simulink model "OFDM_Rx_HW"  (R2020a)
settings: Solver=FixedStepDiscrete  StartTime=0.0  StopTime=inf  RelTol=1e-3
PostLoadFcn:
  | run ./scripts/filter_setup;
InitFcn:
  | % Set parameters
  | fs = 1e6;
  | 
  | % Load all required variables
  | load('variables/read_addr_data');
  | load('variables/read_addr_cp');
  | load('variables/read_addr_pream');
  | load('variables/read_addr_rx');
  | load('variables/pilot');
  | load('variables/sc_index');
  | load('variables/LTSfreq');
  | load('variables/STSfreq');
  | load('variables/LTSread');
  | load('variables/STSread');
undefined symbols (not defined in the file): CIC_fine_Tx
libraries: hdlsllib x11, dspmlti4 x4, xbsIndex_r4 x1, lib_decimaterx x1, lib_ofdmrx x1, lib_ofdmtx x1
settings Model: SimulationMode=accelerator  Creator=njb13206  LastModifiedBy=LDM
settings OptimizationCC: BlockReduction=off  ConditionallyExecuteInputs=off  DefaultParameterBehavior=Inlined
settings DebuggingCC: AlgebraicLoopMsg=error  IntegerOverflowMsg=none  ParameterPrecisionLossMsg=none  IntegerSaturationMsg=none
settings HardwareCC: ProdBitPerPointer=32  ProdBitPerSizeT=32  ProdBitPerPtrDiffT=32  ProdLargestAtomicFloat=None  ProdIntDivRoundTo=Undefined  ProdEndianess=Unspecified  ProdWordSize=32  ProdHWDeviceType=ASIC/FPGA->ASIC/FPGA  TargetBitPerPointer=64  TargetBitPerSizeT=64  TargetBitPerPtrDiffT=64  TargetLongLongMode=on  TargetIntDivRoundTo=Zero  TargetEndianess=LittleEndian  TargetWordSize=64  TargetHWDeviceType=Custom Processor->MATLAB Host Computer  ProdEqTarget=off

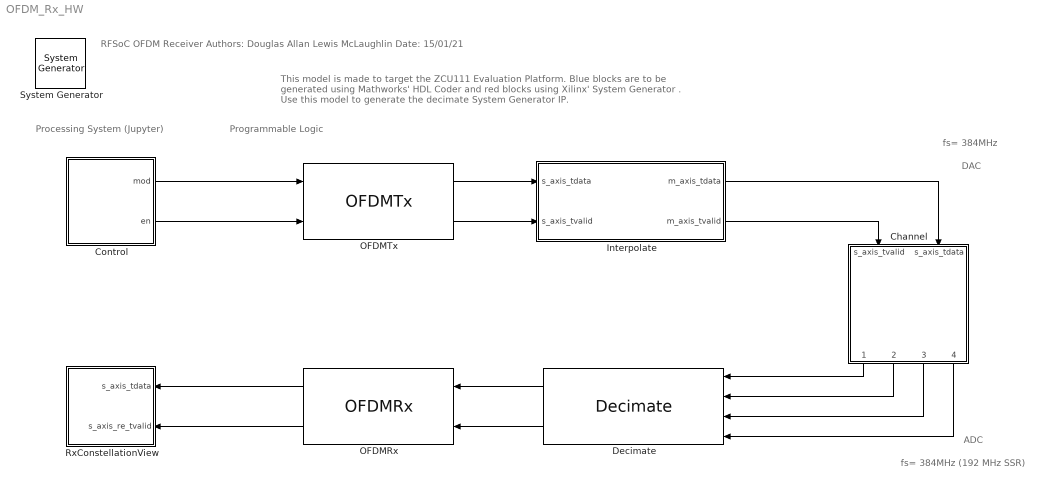
== system OFDM_Rx_HW ==
  note: This model is made to target the ZCU111 Evaluation Platform. Blue blocks are to be generated using Mathworks' HDL Coder and red blocks using Xilinx' System Generator .
      |
      | Use this model to generate the decimate System Generator IP.
  note: Programmable Logic
  note: Processing System (Jupyter)
  note: DAC
  note: fs= 384MHz
  note: ADC
  note: fs= 384MHz (192 MHz SSR)
  note: RFSoC OFDM Receiver
      | Authors: Douglas Allan
      | Lewis McLaughlin
      | Date: 15/01/21
  " System Generator" : xbsIndex_r4/ System Generator  Tag=genX  xilinxfamily=zynquplusRFSOC  part=xczu28dr  speed=-2-e  package=ffvg1517  synthesis_tool=Vivado  clock_wrapper=Clock Enables  directory=C:/Git/rfsoc_ofdm_workspace/models/sys_prj/rx  proj_type=Vivado  Synth_file=Vivado Synthesis Defaults  Impl_file=Vivado Implementation Defaults  testbench=off  simulink_period=1/192e6  sysclk_period=1000/192  dcm_input_clock_period=10  incr_netlist=off  trim_vbits=Everywhere in SubSystem  dbl_ovrd=According to Block Masks  core_generation=According to Block Masks  run_coregen=off  deprecated_control=off  eval_field=0  block_type=sysgen
  Channel : Subsystem
  Control : Subsystem  mask{mod_mask=32QAM, en=on}
      mask prompts: mod_mask "Modulation"; en "Enable"
      mask init:
      | % RF Signal Generator
      | if strcmpi(get_param(gcb, 'mod_mask'), 'BPSK')
      |     mod = 0;
      | elseif strcmpi(get_param(gcb, 'mod_mask'), 'QPSK')
      |     mod = 1;
      | elseif strcmpi(get_param(gcb, 'mod_mask'), '8PSK')
      |     mod = 2;
      | elseif strcmpi(get_param(gcb, 'mod_mask'), '16QAM')
      |     mod = 3;
      | elseif strcmpi(get_param(gcb, 'mod_mask'), '32QAM')
      |     mod = 4;
      | elseif strcmpi(get_param(gcb, 'mod_mask'), '64QAM')
      |     mod = 5;
      | elseif strcmpi(get_param(gcb, 'mod_mask'), '128QAM')
      |     mod = 6;
      | elseif strcmpi(get_param(gcb, 'mod_mask'), '256QAM')
      |     mod = 7;
      | elseif strcmpi(get_param(gcb, 'mod_mask'), '512QAM')
      |     mod = 8;
      | elseif strcmpi(get_param(gcb, 'mod_mask'), '1024QAM')
      |     mod = 9;
      | end
      mask TypeOptions mod_mask: BPSK | QPSK | 8PSK | 16QAM | 32QAM | 64QAM | 128QAM | 256QAM | 512QAM | 1024QAM
      mask DialogControl DescGroupVar Prompt: RF Signal Generator
      mask DialogControl DescTextVar Prompt: Exposes parameters the user can control from Jupyter when running on the target.
      mask DialogControl Container3 Prompt: Control
  Decimate : lib_decimaterx/Decimate  SystemSampleTime=-1  Latency=0  AutoFrameSizeCalculation=off
      link override Up Sample2: sample_ratio=12  copy_samples=off  en=off  latency=1  dbl_ovrd=off
      link override Up Sample2: infoedit="Up samples input data.  Inserted values  can be zeros or copies of the most recent input sample.<br><br>Hardware notes: No hardware is needed if inserted values are copies of the input sample; otherwise, a mux and single bit flip-flop are used."
  Interpolate : Subsystem
  OFDMRx : lib_ofdmrx/OFDMRx  SystemSampleTime=-1  Latency=0  AutoFrameSizeCalculation=off
  OFDMTx : lib_ofdmtx/OFDMTx  SystemSampleTime=-1  Latency=0  AutoFrameSizeCalculation=off
  RxConstellationView : Subsystem
  wires:
  OFDMTx/1 -> Interpolate/1(s_axis_tdata)
  OFDMTx/2 -> Interpolate/2(s_axis_tvalid)
  Channel/1(m00_axis_re_tdata) -> Decimate/1
  Channel/3(m01_axis_im_tdata) -> Decimate/3
  Channel/4(m_axis_im_tvalid) -> Decimate/4
  Channel/2(m_axis_re_tvalid) -> Decimate/2
  Interpolate/1(m_axis_tdata) -> Channel/2(s_axis_tdata)
  Interpolate/2(m_axis_tvalid) -> Channel/1(s_axis_tvalid)
  OFDMRx/2 -> RxConstellationView/2(s_axis_re_tvalid)
  Decimate/1 -> OFDMRx/1
  Decimate/2 -> OFDMRx/2
  OFDMRx/1 -> RxConstellationView/1(s_axis_tdata)
  Control/1(mod) -> OFDMTx/1
  Control/2(en) -> OFDMTx/2

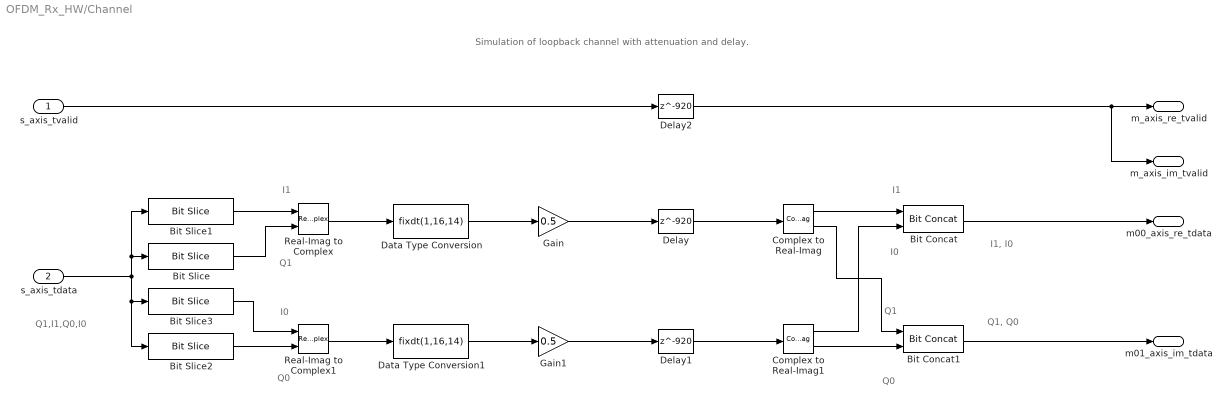
== system OFDM_Rx_HW/Channel ==
  note: Q1, Q0
  note: I1, I0
  note: Q0
  note: I0
  note: Q1
  note: I1
  note: Q1,I1,Q0,I0
  note: Simulation of loopback channel with attenuation and delay.
  note: I1
  note: I0
  note: Q1
  note: Q0
  s_axis_tvalid : Inport
  s_axis_tdata : Inport  Port=2
  Bit Concat : hdlsllib/Logic and Bit Operations/Bit Concat  numInputs=2
  Bit Concat1 : hdlsllib/Logic and Bit Operations/Bit Concat  numInputs=2
  Bit Slice : hdlsllib/Logic and Bit Operations/Bit Slice  lidx=63  ridx=48
      settings: SourceProductBaseCode=SL
  Bit Slice1 : hdlsllib/Logic and Bit Operations/Bit Slice  lidx=47  ridx=32
      settings: SourceProductBaseCode=SL
  Bit Slice2 : hdlsllib/Logic and Bit Operations/Bit Slice  lidx=31  ridx=16
      settings: SourceProductBaseCode=SL
  Bit Slice3 : hdlsllib/Logic and Bit Operations/Bit Slice  lidx=15  ridx=0
      settings: SourceProductBaseCode=SL
  Complex to Real-Imag : ComplexToRealImag
  Complex to Real-Imag1 : ComplexToRealImag
  Data Type Conversion : DataTypeConversion  OutDataTypeStr=fixdt(1,16,14)  ConvertRealWorld=Stored Integer (SI)
  Data Type Conversion1 : DataTypeConversion  OutDataTypeStr=fixdt(1,16,14)  ConvertRealWorld=Stored Integer (SI)
  Delay : Delay  DelayLength=920
  Delay1 : Delay  DelayLength=920
  Delay2 : Delay  DelayLength=920
  Gain : Gain  Gain=0.5  ParamDataTypeStr=double  OutDataTypeStr=fixdt(1,16,14)
  Gain1 : Gain  Gain=0.5  ParamDataTypeStr=double  OutDataTypeStr=fixdt(1,16,14)
  Real-Imag to Complex : RealImagToComplex
  Real-Imag to Complex1 : RealImagToComplex
  m00_axis_re_tdata : Outport  VectorParamsAs1DForOutWhenUnconnected=off
  m_axis_re_tvalid : Outport  Port=2  VectorParamsAs1DForOutWhenUnconnected=off
  m01_axis_im_tdata : Outport  Port=3  VectorParamsAs1DForOutWhenUnconnected=off
  m_axis_im_tvalid : Outport  Port=4  VectorParamsAs1DForOutWhenUnconnected=off
  wires:
  Gain/1 -> Delay/1
  s_axis_tvalid/1 -> Delay2/1
  Delay/1 -> Complex to Real-Imag/1
  Delay2/1 -> m_axis_im_tvalid/1, m_axis_re_tvalid/1
  s_axis_tdata/1 -> Bit Slice1/1, Bit Slice/1, Bit Slice2/1, Bit Slice3/1
  Delay1/1 -> Complex to Real-Imag1/1
  Gain1/1 -> Delay1/1
  Bit Slice/1 -> Real-Imag to Complex/2
  Bit Slice1/1 -> Real-Imag to Complex/1
  Bit Slice2/1 -> Real-Imag to Complex1/2
  Bit Slice3/1 -> Real-Imag to Complex1/1
  Real-Imag to Complex/1 -> Data Type Conversion/1
  Real-Imag to Complex1/1 -> Data Type Conversion1/1
  Complex to Real-Imag1/1 -> Bit Concat/2
  Complex to Real-Imag/1 -> Bit Concat/1
  Complex to Real-Imag1/2 -> Bit Concat1/2
  Complex to Real-Imag/2 -> Bit Concat1/1
  Data Type Conversion/1 -> Gain/1
  Data Type Conversion1/1 -> Gain1/1
  Bit Concat1/1 -> m01_axis_im_tdata/1
  Bit Concat/1 -> m00_axis_re_tdata/1

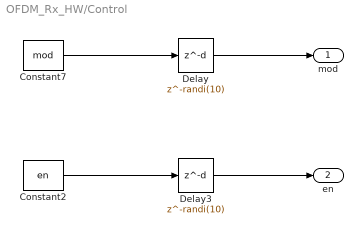
== system OFDM_Rx_HW/Control ==
  Constant2 : Constant  Value=en  OutDataTypeStr=boolean  SampleTime=1/(fs*12)
  Constant7 : Constant  Value=mod  VectorParams1D=off  OutDataTypeStr=uint32  SampleTime=1/(fs*12)
  Delay : Delay  DelayLength=randi(10)
  Delay3 : Delay  DelayLength=randi(10)
  mod : Outport  VectorParamsAs1DForOutWhenUnconnected=off
  en : Outport  Port=2  VectorParamsAs1DForOutWhenUnconnected=off
  wires:
  Delay3/1 -> en/1
  Delay/1 -> mod/1
  Constant7/1 -> Delay/1
  Constant2/1 -> Delay3/1

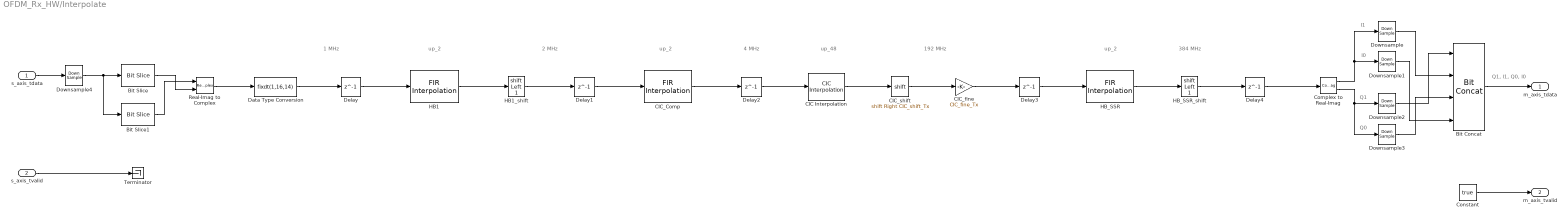
== system OFDM_Rx_HW/Interpolate ==
  note: I0
  note: I1
  note: Q0
  note: Q1
  note: up_2
  note: 4 MHz
  note: 2 MHz
  note: 1 MHz
  note: 384 MHz
  note: 192 MHz
  note: up_2
  note: up_48
  note: up_2
  note: Q1, I1, Q0, I0
  s_axis_tdata : Inport
  s_axis_tvalid : Inport  Port=2
  Bit Concat : hdlsllib/Logic and Bit Operations/Bit Concat  numInputs=4
  Bit Slice : hdlsllib/Logic and Bit Operations/Bit Slice  lidx=15  ridx=0
      settings: SourceProductBaseCode=SL
  Bit Slice1 : hdlsllib/Logic and Bit Operations/Bit Slice  lidx=31  ridx=16
      settings: SourceProductBaseCode=SL
  CIC Interpolation : dspmlti4/CIC Interpolation  filtFrom=Filter object  filtobj=CIC  ftype=Interpolator  R=240  M=1  N=5  filterInternals=Full precision  BPS=[16 16 16 16]  FLPS=0  outputWordLength=32  outputFracLength=0  launchFVT=off  framing=Allow multirate processing  OutputFrames=off
      settings: SourceProductBaseCode=DS
  CIC_Comp : dspmlti4/FIR Interpolation  FilterSource=Dialog parameters  PrivateCoeffs=0  h=WComp.Numerator  L=2  FilterObject=FINTERP  framing=Allow multirate processing  outputBufInitCond=0  roundingMode=Floor  overflowMode=off  firstCoeffMode=Binary point scaling  firstCoeffWordLength=16  firstCoeffFracLength=15  firstCoeffDataTypeStr=fixdt(1,16,15)  firstCoeffMin=[]  firstCoeffMax=[]  firstCoeffLastDataTypeStr=fixdt(1,16,15)  outputMode=Binary point scaling  outputWordLength=16  outputFracLength=14  outputDataTypeStr=fixdt(1,16,14)  outputMin=[]  outputMax=[]  outputLastDataTypeStr=fixdt(1,16,14)
  CIC_fine : Gain  Gain=CIC_fine_Tx  OutDataTypeStr=fixdt(1,16,14)
  CIC_shift : ArithShift  BitShiftNumber=CIC_shift_Tx  BitShiftDirection=Right
  Complex to Real-Imag : ComplexToRealImag
  Constant : Constant  Value=true  SampleTime=2/384e6
  Data Type Conversion : DataTypeConversion  OutDataTypeStr=fixdt(1,16,14)  ConvertRealWorld=Stored Integer (SI)
  Delay{,1..4} (5 alike) : Delay  DelayLength=1
  Downsample : DownSample  phase=1  RateOptions=Allow multirate processing
  Downsample1 : DownSample  RateOptions=Allow multirate processing
  Downsample2 : DownSample  phase=1  RateOptions=Allow multirate processing
  Downsample3 : DownSample  RateOptions=Allow multirate processing
  Downsample4 : DownSample  N=12  phase=5  RateOptions=Allow multirate processing
  HB1 : dspmlti4/FIR Interpolation  FilterSource=Dialog parameters  PrivateCoeffs=0  h=W_HB.Numerator  L=2  FilterObject=FINTERP  framing=Allow multirate processing  outputBufInitCond=0  roundingMode=Floor  overflowMode=off  firstCoeffMode=Binary point scaling  firstCoeffWordLength=16  firstCoeffFracLength=15  firstCoeffDataTypeStr=fixdt(1,16,15)  firstCoeffMin=[]  firstCoeffMax=[]  firstCoeffLastDataTypeStr=fixdt(1,16,15)  outputMode=Binary point scaling  outputWordLength=16  outputFracLength=14  outputDataTypeStr=fixdt(1,16,14)  outputMin=[]  outputMax=[]  outputLastDataTypeStr=fixdt(1,16,14)
  HB1_shift : ArithShift  BitShiftNumber=1  BitShiftDirection=Left
  HB_SSR : dspmlti4/FIR Interpolation  FilterSource=Dialog parameters  PrivateCoeffs=0  h=W_HB_ssr.Numerator  L=2  FilterObject=FINTERP  framing=Allow multirate processing  outputBufInitCond=0  roundingMode=Floor  overflowMode=off  firstCoeffMode=Binary point scaling  firstCoeffWordLength=16  firstCoeffFracLength=15  firstCoeffDataTypeStr=fixdt(1,16,15)  firstCoeffMin=[]  firstCoeffMax=[]  firstCoeffLastDataTypeStr=fixdt(1,16,15)  outputMode=Binary point scaling  outputWordLength=16  outputFracLength=14  outputDataTypeStr=fixdt(1,16,14)  outputMin=[]  outputMax=[]  outputLastDataTypeStr=fixdt(1,16,14)
  HB_SSR_shift : ArithShift  BitShiftNumber=1  BitShiftDirection=Left
  Real-Imag to Complex : RealImagToComplex
  Terminator : Terminator
  m_axis_tdata : Outport
  m_axis_tvalid : Outport  Port=2
  wires:
  CIC_fine/1 -> Delay3/1
  CIC_shift/1 -> CIC_fine/1
  HB_SSR_shift/1 -> Delay4/1
  HB_SSR/1 -> HB_SSR_shift/1
  CIC Interpolation/1 -> CIC_shift/1
  HB1_shift/1 -> Delay1/1
  CIC_Comp/1 -> Delay2/1
  HB1/1 -> HB1_shift/1
  Real-Imag to Complex/1 -> Data Type Conversion/1
  Delay/1 -> HB1/1
  Delay1/1 -> CIC_Comp/1
  Delay2/1 -> CIC Interpolation/1
  Delay3/1 -> HB_SSR/1
  Delay4/1 -> Complex to Real-Imag/1
  Constant/1 -> m_axis_tvalid/1
  Complex to Real-Imag/1 -> Downsample/1, Downsample1/1
  Complex to Real-Imag/2 -> Downsample3/1, Downsample2/1
  Downsample/1 -> Bit Concat/2
  Downsample2/1 -> Bit Concat/1
  Downsample3/1 -> Bit Concat/3
  Downsample1/1 -> Bit Concat/4
  Bit Concat/1 -> m_axis_tdata/1
  s_axis_tvalid/1 -> Terminator/1
  s_axis_tdata/1 -> Downsample4/1
  Downsample4/1 -> Bit Slice1/1, Bit Slice/1
  Bit Slice/1 -> Real-Imag to Complex/2
  Bit Slice1/1 -> Real-Imag to Complex/1
  Data Type Conversion/1 -> Delay/1

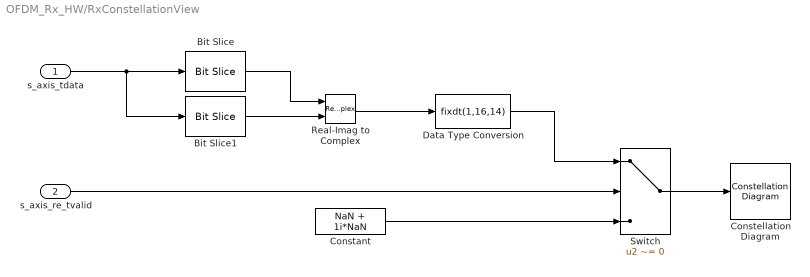
== system OFDM_Rx_HW/RxConstellationView ==
  s_axis_tdata : Inport
  s_axis_re_tvalid : Inport  Port=2
  Bit Slice : hdlsllib/Logic and Bit Operations/Bit Slice  lidx=15  ridx=0
      settings: SourceProductBaseCode=SL
  Bit Slice1 : hdlsllib/Logic and Bit Operations/Bit Slice  lidx=31  ridx=16
      settings: SourceProductBaseCode=SL
  Constant : Constant  Value=NaN + 1i*NaN  OutDataTypeStr=double  SampleTime=-1
  Constellation Diagram : ConstellationDiagram
  Data Type Conversion : DataTypeConversion  OutDataTypeStr=fixdt(1,16,14)  ConvertRealWorld=Stored Integer (SI)
  Real-Imag to Complex : RealImagToComplex
  Switch : Switch  Criteria=u2 ~= 0
  wires:
  Switch/1 -> Constellation Diagram/1
  Constant/1 -> Switch/3
  s_axis_re_tvalid/1 -> Switch/2
  Real-Imag to Complex/1 -> Data Type Conversion/1
  Bit Slice/1 -> Real-Imag to Complex/1
  s_axis_tdata/1 -> Bit Slice1/1, Bit Slice/1
  Bit Slice1/1 -> Real-Imag to Complex/2
  Data Type Conversion/1 -> Switch/1
